simulink model "Correccion_Sist_Fisico"  (R2021a)
settings: Solver=VariableStepAuto  StartTime=0.0  StopTime=inf  RelTol=1e-3
values from neighbouring files (symbols this model uses):
  b_cx = 1*10^6    (= 1000000)    [parametros.m]
  b_cy = 1*10^7    (= 10000000)    [parametros.m]
  b_eq = (b_td+b_tm*(r_t^2))/r_td    (= 10803.6)    [parametros.m]
  b_eqh = 2*(b_hd+b_hm*(r_h^2))/r_hd    (= 23253.3333333)    [parametros.m]
  b_ha = b_eqh/r_h - n_h*w_posh*(J_eqh + 0.5*m_l_*r_hd)/r_h    [parametros.m]
  b_hb = 1*10^8    (= 100000000)    [parametros.m]
  b_hEb = 2.2*10^9    (= 2200000000)    [parametros.m]
  b_t = 90    [parametros.m]
  b_ta = n_t*w_post*(r_td*J_eqt/r_t) - r_td*b_eqt/r_t    [parametros.m]
  b_tb = 5*10^6    (= 5000000)    [parametros.m]
  b_tw = 3*10^3    (= 3000)    [parametros.m]
  b_wu = 150    [parametros.m]
  g = 9.80665    [parametros.m]
  H_c = 2.5    [parametros.m]
  J_eq = (J_td+J_tm_tb*(r_t^2))/r_td    (= 15000)    [parametros.m]
  J_eqh = 2*(J_hd_hEb+J_hm_hb*(r_h^2))/r_hd    (= 48853.3333333)    [parametros.m]
  K_cy = 1.8*10^9    (= 1800000000)    [parametros.m]
  K_hsa = -n_h*(w_posh^2)*(J_eqh + 0.5*m_l_*r_hd)/r_t    [parametros.m]
  K_hsia = -(w_posh^3)*(J_eqh + 0.5*m_l_*r_hd)/r_t    [parametros.m]
  K_tsa = n_t*(w_post^2)*J_eqt*r_td/r_t    [parametros.m]
  K_tsia = (w_post^3)*J_eqt*r_td/r_t    [parametros.m]
  K_tw = 4.8*10^5    (= 480000)    [parametros.m]
  k_wu = 2.36*10^8    (= 236000000)    [parametros.m]
  lh_inicial = 45-yl_inicial    (= 40)    [parametros.m]
  M_c_MAX = 50000 + M_s    (= 65000)    [parametros.m]
  M_real = 10000    [parametros.m]
  M_s = 15000    [parametros.m]
  M_t = 30000    [parametros.m]
  r_h = 22    [parametros.m]
  r_hd = 0.75    [parametros.m]
  r_t = 30    [parametros.m]
  r_td = 0.5    [parametros.m]
  T_hb_MAX = 5*10^4    (= 50000)    [parametros.m]
  T_hEb_MAX = 1.1*10^6    (= 1100000)    [parametros.m]
  T_hm_MAX = 2*10^4    (= 20000)    [parametros.m]
  T_s2 = 5e-3    (= 0.005)    [parametros.m]
  T_tb_MAX = 5*10^3    (= 5000)    [parametros.m]
  T_tm_MAX = 3*10^3    (= 3000)    [parametros.m]
  tau_hm = 1.0e-2    (= 0.01)    [parametros.m]
  tau_tm = 1.0e-2    (= 0.01)    [parametros.m]
  TensionMinima = (M_s*g/2)*0.5    (= 36774.9375)    [parametros.m]
  v_h_MAX_c = +1.5    (= 1.5)    [parametros.m]
  v_t_MAX = +4    (= 4)    [parametros.m]
  v_t_MIN = -4    [parametros.m]
  w_hm_min = pi/4    (= 0.785398163397)    [parametros.m]
  w_tm_min = pi/4    (= 0.785398163397)    [parametros.m]
  xt_inicial = -10    [parametros.m]
  Y_t0 = 45    [parametros.m]
  yl_inicial = 5    [parametros.m]
undefined symbols (not defined in the file or in its folder): DiscIntNeverNeededParam
libraries: simulink x10, dspstat3 x1, vrlib x1
(part 3 of 3)

== stateflow chart Correccion_Sist_Fisico/Chart ==
  note: ---> FINES DE CARRERA:
      |
      | 1. FIN DE CARRERA CARRO:
  state Nivel_1_Apagado
  note: ---> Si el Nivel 1 se encuentra apagodo deberia actuar el Nivel 0
  note: ---> Activado = Freno Energizado = Freno ABIERTO
  note: ---> Desactivado = Freno NO Energizado = Freno CERRADO
  state Nivel_1_Encendido
    state Sobrevelocidad [parallel]
      settings: executionOrder=12
      state CARRO [parallel]
        settings: executionOrder=2
        state Actualizacion_Vel_CARRO
          during:
          dx_t_SobreV = dx_t_ref_man;
        state Analisis_Sobrevelocidad
          entry:
          if (dx_t_ref_man>0)
          dx_t_SobreV = v_t_MAX;
          else
          dx_t_SobreV = v_t_MIN;
          end
        (default) -> Actualizacion_Vel_CARRO
        Actualizacion_Vel_CARRO -> Analisis_Sobrevelocidad : [abs(dx_t_ref_man) > v_t_MAX]
        Analisis_Sobrevelocidad -> Actualizacion_Vel_CARRO : [abs(dx_t_ref_man) <= v_t_MAX]
      state IZAJE [parallel]
        settings: executionOrder=1
        state Actualizacion_Vel_IZAJE
          during:
          dl_h_SobreV = dl_h_ref_man;
        state Analisis_Sobrevelocidad_Pos
          entry:
          dl_h_SobreV = v_h_MAXMIN;
        state Analisis_Sobrevelocidad_Neg
          entry:
          dl_h_SobreV = -v_h_MAXMIN;
        state BAJAR
          entry:
          dl_h_SobreV = v_h_MAX_c*0.1;
        (default) -> Actualizacion_Vel_IZAJE
        Actualizacion_Vel_IZAJE -> Analisis_Sobrevelocidad_Pos [order 1] : [(dl_h_ref_man > v_h_MAXMIN)  && ~sobrecarga ]
        Analisis_Sobrevelocidad_Pos -> Actualizacion_Vel_IZAJE : [(dl_h_ref_man <= v_h_MAXMIN) || sobrecarga ]
        Actualizacion_Vel_IZAJE -> Analisis_Sobrevelocidad_Neg [order 3] : [(dl_h_ref_man < -v_h_MAXMIN)   && ~sobrecarga ]
        Analisis_Sobrevelocidad_Neg -> Actualizacion_Vel_IZAJE : [(dl_h_ref_man >= -v_h_MAXMIN)  || sobrecarga ]
        Actualizacion_Vel_IZAJE -> BAJAR [order 2] : [sobrecarga]
        BAJAR -> Actualizacion_Vel_IZAJE : [~sobrecarga]
    state Fines_de_Carrera [parallel]
      settings: executionOrder=2
      state FIN_DE_CARRERA_CARRO [parallel]
        settings: executionOrder=1
        state Frenar
          entry:
          Detener_CarroFDC = 1;
        state MOVER_CARRO
          during:
          Detener_CarroFDC = 0;
        state No_Frenar
          entry:
          Detener_CarroFDC = 0;
        (default) -> Nivel_1_Encendido.Fines_de_Carrera.FIN_DE_CARRERA_CARRO.No_Frenar
        Nivel_1_Encendido.Fines_de_Carrera.FIN_DE_CARRERA_CARRO.Frenar -> Nivel_1_Encendido.Fines_de_Carrera.FIN_DE_CARRERA_CARRO.MOVER_CARRO [order 2] : [((dx_t_ref_man < 0 && Fin_Der_n) || (dx_t_ref_man > 0 && Fin_Izq_n))]
        Nivel_1_Encendido.Fines_de_Carrera.FIN_DE_CARRERA_CARRO.No_Frenar -> Nivel_1_Encendido.Fines_de_Carrera.FIN_DE_CARRERA_CARRO.Frenar : [Fin_Der_n || Fin_Izq_n]
        Nivel_1_Encendido.Fines_de_Carrera.FIN_DE_CARRERA_CARRO.MOVER_CARRO -> Nivel_1_Encendido.Fines_de_Carrera.FIN_DE_CARRERA_CARRO.Frenar : [(dx_t_ref_man >= 0 && Fin_Der_n) || (dx_t_ref_man <= 0 && Fin_Izq_n) || (~Fin_Der_n && ~Fin_Izq_n) ]
        Nivel_1_Encendido.Fines_de_Carrera.FIN_DE_CARRERA_CARRO.Frenar -> Nivel_1_Encendido.Fines_de_Carrera.FIN_DE_CARRERA_CARRO.No_Frenar [order 1] : [~Fin_Der_n && ~Fin_Izq_n]
      state FIN_DE_CARRERA_IZAJE [parallel]
        settings: executionOrder=2
        state Frenar
          entry:
          Detener_IzajeFDC = 1;
        state MOVER_IZAJE
          during:
          Detener_IzajeFDC = 0;
        state No_Frenar
          entry:
          Detener_IzajeFDC = 0;
        (default) -> Nivel_1_Encendido.Fines_de_Carrera.FIN_DE_CARRERA_IZAJE.No_Frenar
        Nivel_1_Encendido.Fines_de_Carrera.FIN_DE_CARRERA_IZAJE.Frenar -> Nivel_1_Encendido.Fines_de_Carrera.FIN_DE_CARRERA_IZAJE.MOVER_IZAJE [order 2] : [((dl_h_ref_man > 0 && Fin_Sup_n) || (dl_h_ref_man < 0 && Fin_Inf_n))]
        Nivel_1_Encendido.Fines_de_Carrera.FIN_DE_CARRERA_IZAJE.No_Frenar -> Nivel_1_Encendido.Fines_de_Carrera.FIN_DE_CARRERA_IZAJE.Frenar : [Fin_Sup_n || Fin_Inf_n]
        Nivel_1_Encendido.Fines_de_Carrera.FIN_DE_CARRERA_IZAJE.MOVER_IZAJE -> Nivel_1_Encendido.Fines_de_Carrera.FIN_DE_CARRERA_IZAJE.Frenar : [(dl_h_ref_man <= 0 && Fin_Sup_n) || (dl_h_ref_man >= 0 && Fin_Inf_n) || (~Fin_Sup_n && ~Fin_Inf_n) ]
        Nivel_1_Encendido.Fines_de_Carrera.FIN_DE_CARRERA_IZAJE.Frenar -> Nivel_1_Encendido.Fines_de_Carrera.FIN_DE_CARRERA_IZAJE.No_Frenar [order 1] : [~Fin_Sup_n && ~Fin_Inf_n]
    state Frenos [parallel]
      settings: executionOrder=4
      note: % Freno desactivado = Frenando
      state FRENO_CARRO [parallel]
        settings: executionOrder=1
        state No_Frenando
          entry:
          BRK_t = 1;
          Detener_CarroFR = 0;
        state Frenando
          entry:
          BRK_t = 0;
          Detener_CarroFR = 1;
        (default) -> Nivel_1_Encendido.Frenos.FRENO_CARRO.Frenando
        Nivel_1_Encendido.Frenos.FRENO_CARRO.No_Frenando -> Nivel_1_Encendido.Frenos.FRENO_CARRO.Frenando : [(abs(w_tm) < w_tm_min && Freno_Carro_Man) || (Emergencia == 2 && ~Salida_E_C) || sobrecarga || ( dx_t_ref == 0 && dx_t_SobreV == 0) ||  Detener_CarroFDC || (dx_t_ref * dx_t_ref_man < 0) ]
        Nivel_1_Encendido.Frenos.FRENO_CARRO.Frenando -> Nivel_1_Encendido.Frenos.FRENO_CARRO.No_Frenando : [Tmt_disp && ~Freno_Carro_Man && (Emergencia == 0 || Salida_E_C) && ~sobrecarga && ( dx_t_ref ~= 0 || dx_t_SobreV ~= 0) && ~Detener_CarroFDC && (dx_t_ref * dx_t_ref_man >= 0)]
      state FRENO_IZAJE [parallel]
        settings: executionOrder=2
        state No_Frenando
          entry:
          BRK_h = 1;
          Detener_IzajeFR = 0;
        state Frenando
          entry:
          BRK_h = 0;
          Detener_IzajeFR = 1;
        (default) -> Nivel_1_Encendido.Frenos.FRENO_IZAJE.Frenando
        Nivel_1_Encendido.Frenos.FRENO_IZAJE.No_Frenando -> Nivel_1_Encendido.Frenos.FRENO_IZAJE.Frenando : [(abs(w_hm) < w_hm_min && Freno_Izaje_Man) || (Emergencia == 3 && ~Salida_E_I)  || (sobrecarga && dl_h_ref <= 0) || ( dl_h_ref == 0 && dl_h_SobreV == 0) || Detener_IzajeFDC || ~Cable_Tenso || (45-l_h < y_obstaculo-0.15 && dl_h_ref_man >= 0) || (dl_h_ref * dl_h_ref_man < 0)]
        Nivel_1_Encendido.Frenos.FRENO_IZAJE.Frenando -> Nivel_1_Encendido.Frenos.FRENO_IZAJE.No_Frenando : [Tmh_disp && ~Freno_Izaje_Man && (Emergencia == 0 || Salida_E_I) && (~sobrecarga || sobrecarga && dl_h_ref > 0) && ( dl_h_ref ~= 0 || dl_h_SobreV ~= 0) && ~Detener_IzajeFDC && Cable_Tenso && (45-l_h >= y_obstaculo-0.15 || dl_h_ref_man < 0) && (dl_h_ref * dl_h_ref_man >= 0)]
      state FRENO_EMERGENCIA [parallel]
        settings: executionOrder=3
        state No_Frenando
          entry:
          BRK_hE = 1;
        state Frenando
          entry:
          BRK_hE = 0;
        (default) -> Nivel_1_Encendido.Frenos.FRENO_EMERGENCIA.Frenando
        Nivel_1_Encendido.Frenos.FRENO_EMERGENCIA.No_Frenando -> Nivel_1_Encendido.Frenos.FRENO_EMERGENCIA.Frenando : [~Grua_Encendida || (45-l_h < y_obstaculo-0.2 && dl_h_ref_man >= 0)]
        Nivel_1_Encendido.Frenos.FRENO_EMERGENCIA.Frenando -> Nivel_1_Encendido.Frenos.FRENO_EMERGENCIA.No_Frenando : [Grua_Encendida && (45-l_h > y_obstaculo-0.2 || dl_h_ref_man < 0)]
    state Sobrecarga [parallel]
      settings: executionOrder=7
      note: SI HAY SOBRECARGA SOLO SE PUEDE BAJAR MANUALMENTE
      state CON_SOBRECARGA
        entry:
        sobrecarga = 1;
      state SIN_SOBRECARGA
        entry:
        sobrecarga = 0;
      (default) -> SIN_SOBRECARGA
      SIN_SOBRECARGA -> CON_SOBRECARGA : [M_cX > M_c_MAX && MasaFija && TLK]
      CON_SOBRECARGA -> SIN_SOBRECARGA : [M_cX < M_c_MAX && MasaFija && ~TLK]
    state Twistlocks [parallel]
      settings: executionOrder=3
      note: SE ACTIVA EL TLK SI EL OPERARIO LO DESEA Y
          | ADEMAS LA TENSION EN EL CABLE ES 0 (spreader apoyado)
      state TLK_ABIERTO
        entry:
        TLK = 0;
        y_obstaculo = 0;
        during:
        y_obstaculo = Y_co;
      state TLK_CERRADO
        entry:
        TLK = 1;
        during:
        y_obstaculo = Y_co + 2.5;
      (default) -> TLK_ABIERTO
      TLK_CERRADO -> TLK_ABIERTO : [~Activar_TLK && ~Cable_Tenso && TLK]
      TLK_ABIERTO -> TLK_CERRADO : [Activar_TLK && ~Cable_Tenso && ~TLK]
    state Senal_Vida [parallel]
      settings: executionOrder=9
      state Pulso_alto
        entry:
        Vida=1;
      state Pulso_bajo
        entry:
        Vida=0;
      (default) -> Pulso_bajo
      Pulso_bajo -> Pulso_alto : after(500,msec)
      Pulso_alto -> Pulso_bajo : after(10,msec)
    state Deteccion_Cable_Flojo [parallel]
      settings: executionOrder=5
      state CABLE_TENSO
        entry:
        Cable_Tenso = 1;
      state CABLE_FLOJO
        entry:
        Cable_Tenso = 0;
      (default) -> CABLE_TENSO
      CABLE_FLOJO -> CABLE_TENSO : [dl_h_ref_man < 0 || F_hw > TensionMinima ]
      CABLE_TENSO -> CABLE_FLOJO : [dl_h_ref_man >= 0 && F_hw <= TensionMinima]
    state Control_De_Balanceo [parallel]
      settings: executionOrder=6
      state ACTIVADO
        entry:
        BAC = 1;
      state DESACTIVADO
        entry:
        BAC = 0;
      (default) -> DESACTIVADO
      ACTIVADO -> DESACTIVADO : [~Balanceo || Emergencia ~=0]
      DESACTIVADO -> ACTIVADO : [Balanceo && Emergencia == 0]
    state MOVER_GRUA_ESTADO_EMERGENCIA_IZAJE [parallel]
      settings: executionOrder=10
      state MOVER_IZAJE
        entry:
        Salida_E_I = 1;
      state EMERGENCIA_IZAJE
        entry:
        Salida_E_I = 0;
      state NORMAL
        entry:
        Salida_E_I = 0;
      (default) -> NORMAL
      EMERGENCIA_IZAJE -> Nivel_1_Encendido.MOVER_GRUA_ESTADO_EMERGENCIA_IZAJE.MOVER_IZAJE [order 2] : [(dl_h_ref_man > 0 && Fin_Sup_u) || (dl_h_ref_man < 0 && Fin_Inf_u)]
      NORMAL -> EMERGENCIA_IZAJE : [Emergencia == 3]
      EMERGENCIA_IZAJE -> NORMAL [order 1] : [Emergencia == 0]
      Nivel_1_Encendido.MOVER_GRUA_ESTADO_EMERGENCIA_IZAJE.MOVER_IZAJE -> EMERGENCIA_IZAJE : [(dl_h_ref_man <= 0 && Fin_Sup_u) || (dl_h_ref_man >= 0 && Fin_Inf_u) || Emergencia == 0]
    state MOVER_GRUA_ESTADO_EMERGENCIA_CARRO [parallel]
      settings: executionOrder=11
      state MOVER_CARRO
        entry:
        Salida_E_C = 1;
      state INICIO
        entry:
        Salida_E_C = 0;
      state ESPERA
        Salida_E_C = 0;
      (default) -> INICIO
      ESPERA -> Nivel_1_Encendido.MOVER_GRUA_ESTADO_EMERGENCIA_CARRO.MOVER_CARRO [order 2] : [(dx_t_ref_man < 0 && Fin_Der_u) || (dx_t_ref_man > 0 && Fin_Izq_u)]
      INICIO -> ESPERA : [Emergencia == 2]
      Nivel_1_Encendido.MOVER_GRUA_ESTADO_EMERGENCIA_CARRO.MOVER_CARRO -> ESPERA : [(dx_t_ref_man >= 0 && Fin_Der_u) || (dx_t_ref_man <= 0 && Fin_Izq_u) || Emergencia == 0]
      ESPERA -> INICIO [order 1] : [Emergencia == 0]
    state Modo [parallel]
      settings: executionOrder=8
      state MANUAL
        entry:
        Modo_Manual = 1;
        IteracionTerminada = 0;
        state Carro [parallel]
          settings: executionOrder=1
          state Operacion_Normal
            during:
            dx_t_ref = calcular_velocidad_maximaC(dx_t_SobreV);
          state sobrecarga_Carro
            entry:
            dx_t_ref = 0;
            calcular_velocidad_maximaC(0);
          state Analisis_FDC_D
            during:
            dx_t_ref = calcular_velocidad_maximaC(dx_t_SobreV*(50-x_td)/10);
          state Analisis_FDC_I
            during:
            dx_t_ref = calcular_velocidad_maximaC(dx_t_SobreV*(30+x_td)/10);
          state detener_carro
            entry:
            dx_t_ref = 0;
            calcular_velocidad_maximaC(0);
          (default) -> Nivel_1_Encendido.Modo.MANUAL.Carro.Operacion_Normal
          Analisis_FDC_D -> Nivel_1_Encendido.Modo.MANUAL.Carro.Operacion_Normal : [Detener_CarroFR || Detener_CarroFDC || dx_t_ref_man < 0]
          Nivel_1_Encendido.Modo.MANUAL.Carro.Operacion_Normal -> sobrecarga_Carro [order 1] : [sobrecarga]
          sobrecarga_Carro -> Nivel_1_Encendido.Modo.MANUAL.Carro.Operacion_Normal : [~sobrecarga]
          Nivel_1_Encendido.Modo.MANUAL.Carro.Operacion_Normal -> Analisis_FDC_D [order 3] : [x_td >=40 && dx_t_ref_man > 0 && ~Detener_CarroFR && ~Detener_CarroFDC && ~Fin_Der_n && ~Fin_Izq_n]
          Analisis_FDC_I -> Nivel_1_Encendido.Modo.MANUAL.Carro.Operacion_Normal : [Detener_CarroFR || Detener_CarroFDC || dx_t_ref_man > 0]
          Nivel_1_Encendido.Modo.MANUAL.Carro.Operacion_Normal -> detener_carro [order 2] : [Detener_CarroFR || Detener_CarroFDC ]
          Nivel_1_Encendido.Modo.MANUAL.Carro.Operacion_Normal -> Analisis_FDC_I [order 4] : [x_td <=-20 && dx_t_ref_man < 0 && ~Detener_CarroFR && ~Detener_CarroFDC]
          detener_carro -> Nivel_1_Encendido.Modo.MANUAL.Carro.Operacion_Normal : [~Detener_CarroFR  && ~Detener_CarroFDC ]
        state Izaje [parallel]
          settings: executionOrder=2
          note: dl_h_ref_man se refiere a longitud del cable. Si es >0, se tiene mayor longitud de cable y la carga baja. Si es <0 la longitud disminuye y la carga baja. El 5 en FDC_ARRIBA es una medida de seguridad. En estimacion de masa se limita la velocidad al 10%.
          state Operacion_Normal
            during:
            dl_h_ref = calcular_velocidad_maxima_I(dl_h_SobreV, MasaFija);
          state sobrecarga_Izaje
            during:
            if (dl_h_ref_man>0)
            dl_h_ref = calcular_velocidad_maxima_I(dl_h_SobreV, MasaFija);
            else
            dl_h_ref = 0;
            calcular_velocidad_maxima_I(0, MasaFija);
            end
          state Analisis_FDC_ARRIBA
            during:
            dl_h_ref = calcular_velocidad_maxima_I(dl_h_SobreV*(l_h-5)/5, MasaFija);
          state Analisis_FDC_ABAJO
            during:
            dl_h_ref = calcular_velocidad_maxima_I(dl_h_SobreV*(65-l_h)/10, MasaFija);
          state detener_Izaje
            entry:
            dl_h_ref = 0;
            calcular_velocidad_maxima_I(0, MasaFija);
          state Analisis_ESTIMACION_MASA
            during:
            dl_h_ref = calcular_velocidad_maxima_I(dl_h_SobreV, MasaFija)*0.1;
          state Analisis_OBSTACULO
            during:
            dl_h_ref = calcular_velocidad_maxima_I(dl_h_SobreV*(45-y_obstaculo-l_h+0.2)/5, MasaFija);
          (default) -> Nivel_1_Encendido.Modo.MANUAL.Izaje.Operacion_Normal
          Analisis_FDC_ARRIBA -> Nivel_1_Encendido.Modo.MANUAL.Izaje.Operacion_Normal : [Detener_IzajeFR || Detener_IzajeFDC || dl_h_ref_man > 0]
          Nivel_1_Encendido.Modo.MANUAL.Izaje.Operacion_Normal -> sobrecarga_Izaje [order 1] : [sobrecarga]
          Nivel_1_Encendido.Modo.MANUAL.Izaje.Operacion_Normal -> Analisis_FDC_ARRIBA [order 4] : [l_h <=10 && dl_h_ref_man < 0 && ~Detener_IzajeFR && ~Detener_IzajeFDC]
          sobrecarga_Izaje -> Nivel_1_Encendido.Modo.MANUAL.Izaje.Operacion_Normal : [~sobrecarga]
          Analisis_FDC_ABAJO -> Nivel_1_Encendido.Modo.MANUAL.Izaje.Operacion_Normal : [Detener_IzajeFR || Detener_IzajeFDC  || dl_h_ref_man < 0]
          Nivel_1_Encendido.Modo.MANUAL.Izaje.Operacion_Normal -> Analisis_FDC_ABAJO [order 5] : [l_h >=55 && dl_h_ref_man > 0 && ~Detener_IzajeFR && ~Detener_IzajeFDC]
          Analisis_ESTIMACION_MASA -> Nivel_1_Encendido.Modo.MANUAL.Izaje.Operacion_Normal : [MasaFija || sobrecarga || Detener_IzajeFR || Detener_IzajeFDC]
          Nivel_1_Encendido.Modo.MANUAL.Izaje.Operacion_Normal -> detener_Izaje [order 2] : [(Detener_IzajeFR || Detener_IzajeFDC) && ~sobrecarga]
          detener_Izaje -> Nivel_1_Encendido.Modo.MANUAL.Izaje.Operacion_Normal : [(~Detener_IzajeFR && ~Detener_IzajeFDC) || sobrecarga]
          Nivel_1_Encendido.Modo.MANUAL.Izaje.Operacion_Normal -> Analisis_ESTIMACION_MASA [order 6] : [~MasaFija && TLK && ~Detener_IzajeFR && ~Detener_IzajeFDC && Cable_Tenso]
          Analisis_OBSTACULO -> Nivel_1_Encendido.Modo.MANUAL.Izaje.Operacion_Normal : [Detener_IzajeFR || Detener_IzajeFDC  || dl_h_ref_man < 0]
          Nivel_1_Encendido.Modo.MANUAL.Izaje.Operacion_Normal -> Analisis_OBSTACULO [order 3] : [(y_obstaculo+5) >= (45-l_h) && dl_h_ref_man > 0 && ~Detener_IzajeFR && ~Detener_IzajeFDC]
      state AUTOMATICO
        entry:
        Modo_Manual = 0;
        esperando_estabilizacion=true;
        punto_muelle = [-20, 0];
        trayectoria = 0;
        punto_carga = [-10, 5];
        punto_descarga = [-15, 5];
        [contenedor_posiciones, y_max] = actualizar_contenedores(contenedor_pos_iniciales, -10, 10);
      (default) -> MANUAL
      MANUAL -> AUTOMATICO : [Cambiar_Modo && ~IteracionTerminada]
      AUTOMATICO -> MANUAL : [~Cambiar_Modo && IteracionTerminada || Emergencia || dx_t_ref_man ~= 0 || dl_h_ref_man ~= 0]
    state OBSTACULOS [parallel]
      entry:
      [contenedor_posiciones, y_max] = actualizar_contenedores(contenedor_pos_iniciales, -10, 10); % Pongo valor random para q me devuelva
      matriz_Y_co = calculo_matriz_yc0(contenedor_posiciones)                                                        % el y_max y no hacer otra funcion
      settings: executionOrder=1
      state ACTUALIZACION_CONTENEDORES [parallel]
        settings: executionOrder=1
        state Verificar
        state Carga
          entry:
          y_actual = pos_y_actual(l_h, TLK);
          [contenedor_posiciones, y_max] = actualizar_contenedores(contenedor_posiciones, x_td, y_actual);
          matriz_Y_co = calculo_matriz_yc0(contenedor_posiciones);
        state Descarga
          entry:
          % Por ahora no hace nada, va a servir para los otros modos
        (default) -> Verificar
        Verificar -> Carga [order 1] : [~Cable_Tenso &&  Activar_TLK && ~TLK ]
        Carga -> Verificar : [Cable_Tenso && MasaFija]
        Verificar -> Descarga [order 2] : [Cable_Tenso &&  ~Activar_TLK && TLK ]
        Descarga -> Verificar : [~Cable_Tenso]
      state CALCULAR_YCO [parallel]
        settings: executionOrder=2
        state Calculo_YC0
          during:
          Y_co = obtener_Y_c0(matriz_Y_co, x_td);
        (default) -> Calculo_YC0
  (default) -> Nivel_1_Apagado
  Nivel_1_Apagado -> Nivel_1_Encendido : [Alimentacion]
  Nivel_1_Encendido -> Nivel_1_Apagado : [~Alimentacion]
  data: dx_manual function_input; v_max_carro function_output; dh_manual function_input; v_max_izaje function_output; Enclave function_input; contenedor_pos function_output; contenedor_pos function_input; pos_x function_input; pos_y function_input; y_superior function_output; obstaculos function_input; punto_inicial function_input; punto_final function_input; Carga_Descarga_ function_input; perfil_trayectoria function_output; sx function_output; sy function_output; contenedor_pos function_output; contenedor_pos function_input; pos_x function_input; pos_y function_input; y_superior function_output; matriz_yc0 function_output; contenedor_pos function_input; matriz_yc0 function_input; yc0 function_output; xtd function_input; l function_input; tlk function_input; pos_y function_output; Alimentacion input; Fin_Der_n input; Fin_Izq_n input; Fin_Sup_n input; Fin_Inf_n input; BRK_t output; BRK_h output; BRK_hE output; Vida output size=1; Emergencia input; Grua_Encendida input; dx_t_ref_man input; dl_h_ref_man input; w_tm input; w_hm input; Freno_Carro_Man input; Freno_Izaje_Man input; Balanceo input; x_td input; l_h input; MasaFija input; Activar_TLK input; M_cX input; dx_t_ref output =0; dl_h_ref output =0; BAC output; TLK output size=1; v_t_MAX parameter; v_t_MIN parameter; Tmt_disp input; w_tm_min parameter; w_hm_min parameter; Tmh_disp input; F_hw input; v_h_MAX_c parameter; Modo_Manual output size=1; Detener_Carro local; Detener_Izaje local; Cable_Tenso local; dx_t_SobreV local =0; dl_h_SobreV local =0; sobrecarga local; M_c_MAX parameter; TensionMinima parameter; v_h_MAXMIN input; Detener_IzajeFDC local; Detener_CarroFDC local; Detener_CarroFR local; Detener_IzajeFR local; Fin_Sup_u input; Fin_Inf_u input; Cambio_Modo input; Fin_Izq_u input; Fin_Der_u input; Salida_E_C local; Salida_E_I local; bajar_sobrecarga local; y_obstaculo local; esperando_estabilizacion local; punto_limite local; punto_muelle local; trayectoria_y local; perfil_vel_x local; punto_inicial local; posicion_final local; perfil_vel_y local; Cambiar_Modo local; cant_puntos_discretizacion local; y_l local; y_sup local; it local; posicion_y_actual local size=1 =yl_inicial; y_max local; y_actual local; matriz_Y_co local size=1,16; contenedor_posiciones local size=18,16; contenedor_pos_iniciales input; Y_co output size=1
  function v_max_carro = calcular_velocidad_maximaC(dx_manual):
    | function v_max_carro = calcular_velocidad_maximaC(dx_manual)
    | 
    | %--------------------------------------------------------------------------%
    | %---------------------Declaracion variables PERSISTENT---------------------% 
    | %--------------------------------------------------------------------------%
    |             % --> Persistent: local variable in a function that retains its 
    |                             % value in memory between calls to the function
    |     persistent dx_t_ref_manual_anterior;
    |     a_max_carro = 1;     % m/s^2 (aceleracion max para el subsistema carro)
    |     dt = 0.02;           % 20 ms (tiempo de muestreo del statechart)
    |     
    | %--------------------------------------------------------------------------%
    | %------------------Inicialización de variables PERSISTENT------------------% 
    | %--------------------------------------------------------------------------%
    | 
    |     if isempty(dx_t_ref_manual_anterior)
    |         dx_t_ref_manual_anterior = 0;
    |     end
    |     
    | %--------------------------------------------------------------------------%
    | %-----------------------------Lógica principal-----------------------------%
    | %--------------------------------------------------------------------------%
    | % La idea es que el sistema siempre vaya a la maxima velocidad que pueda.
    | % Para eso se utiliza la aceleracion maxima para el subsistema carro en
    | % caso de que la velocidad de referencia no sea lo suficientemente grande.
    | % Si la velocidad supera la velocidad maxima, esta se limita al maximo
    | % permitido.
    |     if (dx_manual == 0)
    |         v_max_carro_aux = 0;
    |     else
    |         if abs(dx_manual) >= abs(dx_t_ref_manual_anterior)
    |             if dx_manual > 0                                                    % Aceleracion +
    |                 v_max = a_max_carro * dt + dx_t_ref_manual_anterior;
    |                 v_max_carro_aux = max(v_max, dx_manual);
    |             else                                                                % Aceleracion -
    |                 v_max = -a_max_carro * dt + dx_t_ref_manual_anterior;
    |                 v_max_carro_aux = min(v_max, dx_manual);
    |             end
    |         elseif dx_manual < dx_t_ref_manual_anterior                             % Desaceleracion -
    |             v_max = -a_max_carro * dt + dx_t_ref_manual_anterior;
    |             v_max_carro_aux = min(v_max, dx_manual);
    |         else                                                                    % Desaceleracion +
    |             v_max = a_max_carro * dt + dx_t_ref_manual_anterior;
    |             v_max_carro_aux = max(v_max, dx_manual);
    |         end
    | 
    |         if abs(v_max_carro_aux) > 4
    |             if v_max_carro_aux > 0
    |                 v_max_carro_aux = 4;
    |             else
    |                 v_max_carro_aux = -4;
    |             end
    |         end
    |     end
    |     v_max_carro = v_max_carro_aux;
    | 
    |     dx_t_ref_manual_anterior = v_max_carro;
    | end
  function v_max_izaje =   calcular_velocidad_maxima_I(dh_manual, Enclave):
    | function v_max_izaje =   calcular_velocidad_maxima_I(dh_manual, Enclave) % CT es Cable Tenso
    | 
    | %--------------------------------------------------------------------------%
    | %---------------------Declaracion variables PERSISTENT---------------------% 
    | %--------------------------------------------------------------------------%
    |             % --> Persistent: local variable in a function that retains its 
    |                             % value in memory between calls to the function
    |     persistent dy_href_manual_ant;
    |     persistent a_max_y;  % m/s^2
    |     persistent dt;       % 20 ms (tiempo de muestreo del statechart)
    |     
    | %--------------------------------------------------------------------------%
    | %------------------Inicialización de variables PERSISTENT------------------% 
    | %--------------------------------------------------------------------------%
    | 
    |     if isempty(dy_href_manual_ant)
    |         dy_href_manual_ant = 0;
    |     end
    |     if isempty(a_max_y)
    |         a_max_y = 0.75;  % m/s^2
    |     end
    |     if isempty(dt)
    |         dt = 0.02;       % 20 ms (tiempo de muestreo del statechart)
    |     end
    |     
    | %--------------------------------------------------------------------------%
    | %-----------------------------Lógica principal-----------------------------%
    | %--------------------------------------------------------------------------%
    | % La idea es que el sistema siempre vaya a la maxima velocidad que pueda.
    | % Para eso se utiliza la aceleracion maxima para el subsistema carro en
    | % caso de que la velocidad de referencia no sea lo suficientemente grande.
    | % Si la velocidad supera la velocidad maxima, esta se limita al maximo
    | % permitido.
    |     if (dh_manual ==0)
    |         v_max_izaje_aux = 0;
    |     else
    |         if abs(dh_manual) >= abs(dy_href_manual_ant)
    |             if dh_manual > 0
    |                 v_max = a_max_y * dt + dy_href_manual_ant;
    |                 v_max_izaje_aux = max(v_max, dh_manual);
    |             else
    |                 v_max = -a_max_y * dt + dy_href_manual_ant;
    |                 v_max_izaje_aux = min(v_max, dh_manual);
    |             end
    |         else
    |             if dh_manual < dy_href_manual_ant
    |                 v_max = -a_max_y * dt + dy_href_manual_ant;
    |                 v_max_izaje_aux = min(v_max, dh_manual);
    |             else
    |                 v_max = a_max_y * dt + dy_href_manual_ant;
    |                 v_max_izaje_aux = max(v_max, dh_manual);
    |             end
    |         end
    | 
    |         if Enclave == 1      % Hay carga, velocidad maxima 1.5 m/s
    |             if abs(v_max_izaje_aux) > 1.5
    |                 if v_max_izaje_aux > 0
    |                     v_max_izaje_aux = 1.5;
    |                 else
    |                     v_max_izaje_aux = -1.5;
    |                 end
    |             end
    |         else                % No hay carga, velocidad maxima 3 m/s
    |             if abs(v_max_izaje_aux) > 3
    |                 if v_max_izaje_aux > 0
    |                     v_max_izaje_aux = 3;
    |                 else
    |                     v_max_izaje_aux = -3;
    |                 end
    |             end
    |         end
    |     end
    |     v_max_izaje = v_max_izaje_aux;
    |     dy_href_manual_ant = v_max_izaje;
    | 
    | end
  function [contenedor_pos, y_superior] = actualizar_contenedores(contenedor_pos, pos_x, pos_y):
    | function [contenedor_pos, y_superior] = actualizar_contenedores(contenedor_pos, pos_x, pos_y)
    |     for columna = 1:size(contenedor_pos, 2)
    |         cantidad_contenedores_columna = sum(contenedor_pos(:,columna));
    |         if cantidad_contenedores_columna ~= 0 % Es decir si quedan contenedores en esa columna
    |             pos_x_izq_contenedor = 2.5 + (columna - 1) * 3;
    |             pos_x_der_contenedor = pos_x_izq_contenedor + 2.5;
    |             tolerancia = 0.2;
    |             pos_y_superior_contenedor = cantidad_contenedores_columna * 2.5 + tolerancia;
    |             if pos_x > pos_x_izq_contenedor && pos_x < pos_x_der_contenedor && pos_y < pos_y_superior_contenedor 
    |                 contenedor_pos(cantidad_contenedores_columna, columna) = 0;
    |                 break;
    |             end
    |         end
    |     end
    |     unos_por_columna = sum(contenedor_pos); % Me da la suma de cada columna
    |     max_contenedores = max(unos_por_columna); % Busco el máximo de la suma de cada columna
    |     
    |     coef_seguridad = 5;
    |     y_superior = max_contenedores*2.5 + coef_seguridad;
    | end
  function [perfil_trayectoria, sx, sy]  = generar_Trayectoria2(obstaculos, punto_inicial, punto_final, Carga_Descarga_):
    | function [perfil_trayectoria, sx, sy]  = generar_Trayectoria2(obstaculos, punto_inicial, punto_final, Carga_Descarga_) 
    | 
    | %===================================================PERFIL DE VELOCIDAD
    |     %________________Aceleraciones y velocidades
    |     
    | 
    |     perfil_vel_x = [0];
    |     perfil_vel_y = [];
    |     
    |     amax_Y = 0.75;
    |     vmax_Y = 3;
    |     vmax_X = 4;
    |     amax_X = 1;
    |     
    |     
    | %===================================================PERFIL DE TRAYECTORIA
    |     %________________Definir inicio contenedores y el factor de seguridad
    |     factor_seguridad = 3;
    |     inicio_contenedores = [2.5, -20];
    |     contador = 0;
    |     
    |     separacion_contenedores = 0.5;
    |     pared_barco = zeros(length(obstaculos(:,1)),1);
    |     pared_barco(1:2, 1) = [1, 1];
    |     obstaculos = [pared_barco, obstaculos];
    |     
    |     %________________Definir las dimensiones de los contenedores y el incremento de altura y posición
    |     ancho_contenedor = 2.5;
    |     alto_contenedor = 2.5;
    |     incremento_altura = 2;
    |     incremento_posicion = 0.625;
    |     incremento_altura_vuelta = 1;
    |     incremento_altura_bajada = 3;
    |     punto_final_aux = 0;
    |     
    |     
    |     % Inicializar el perfil de trayectoria como un vector vacío
    |     perfil_trayectoria = [punto_inicial];
    | 
    |     % Verificar cual es el obstáculo más alto
    |     obstaculo_mas_alto = max(sum(obstaculos, 1));
    | 
    |     % Calcular la altura del obstáculo más alto en metros
    |     if Carga_Descarga_ == 0
    |         altura_obstaculo_mas_alto = obstaculo_mas_alto * alto_contenedor + factor_seguridad*2 + inicio_contenedores(1, 2);
    |     else
    |         posicion = encontrar_posicion(punto_inicial, obstaculos);
    |         if posicion > 1
    |             contenedores_por_fila = cant_contenedores(obstaculos(:,posicion-1));
    |             altura_obstaculo_mas_alto = contenedores_por_fila * alto_contenedor + factor_seguridad*2 + inicio_contenedores(1, 2);
    |         elseif posicion == 1
    |             contenedores_por_fila = cant_contenedores(obstaculos(:,posicion+1));
    |             altura_obstaculo_mas_alto = contenedores_por_fila * alto_contenedor + factor_seguridad*2 + inicio_contenedores(1, 2);
    |         else
    |             altura_obstaculo_mas_alto = 7;
    |         end
    |     end
    | 
    |     if (punto_inicial(1, 1) < punto_final(1,1))
    |         disp('hola')
    |         punto_final = modificacion_punto_final(obstaculos,punto_final,  ancho_contenedor,alto_contenedor, factor_seguridad, separacion_contenedores);
    |     
    |         % Buscar una línea que una el punto inicial con un punto P2 ubicado en x en la pared del barco y con una altura igual a la del obstáculo más alto
    |         P2 = [0 + ancho_contenedor/2, altura_obstaculo_mas_alto]
    | 
    |         % Verificar si la línea colisiona con el perfil de obstáculos
    |         
    |         
    |         dy = P2(1,2) - punto_inicial(1,2);
    |         dx = P2(1,1) - punto_inicial(1,1);
    |         Tx1 = vmax_X/amax_X                                                 % TIEMPO HASTA VELOCIDAD MAX
    |         Tx3 = (abs(dx) - 0.5*(Tx1^2)*amax_X)/vmax_X
    |         if (Tx3>0)
    |             Tx = Tx1 + Tx3;
    |         else
    |             Tx = Tx1;
    |         end
    |         Ty1 = vmax_Y/amax_Y;
    |         Ty3 = (abs(dy) - 2*0.5*(Ty1^2)*amax_Y)/vmax_Y;
    |         Ty = 2*Ty1 + Ty3  % TIEMPO PERFIL TRAPEZOIDAL
    |         Tx
    |         if(Tx == Ty)
    |             disp('');
    |             colision = verificar_colision_SUBIDA_IDA(obstaculos, punto_inicial, P2, ancho_contenedor, alto_contenedor, factor_seguridad);
    |         else                                                                % SIEMPRE TY VA A SER MAS GRANDE
    |             T = Ty - Tx
    |             
    |             if T <= Ty1
    |                 dy_aux  = 0.5*amax_Y*(T^2);
    |             elseif T > Ty1 && T<= Ty1 + Ty3
    |                 dy_aux = 0.5*amax_Y*(Ty1^2) + vmax_Y*(T-Ty1);
    |             else 
    |                 dy_aux = 0.5*amax_Y*(Ty1^2) + vmax_Y*(Ty3) + vmax_Y*(T - Ty1 - Ty3) - 0.5*amax_Y*((T - Ty1 - Ty3)^2);
    |             end
    |             colision = verificar_colision_SUBIDA_IDA(obstaculos, punto_inicial, P2, ancho_contenedor, alto_contenedor, factor_seguridad);
    |             
    |             if true
    |                 perfil_vel_y = [perfil_vel_y, linspace(0, vmax_Y, Ty1/0.005), linspace(vmax_Y, vmax_Y, Ty3/0.005), linspace(vmax_Y, 0, Ty1/0.005)];
    |                 if (Tx3>=0)
    |                     disp('Hola')
    |                      perfil_vel_x = [perfil_vel_x, linspace(0, 0, T/0.005), linspace(0, vmax_X, (Tx1)/0.005), linspace(vmax_X, vmax_X, (Tx3)/0.005)];
    |                 else
    |                      perfil_vel_x = [perfil_vel_x, linspace(0, 0, T/0.005), linspace(0, vmax_X, (Tx)/0.005)];
    |                 end
    |                 
    |                 sx = punto_inicial(1,1);
    |                 sy = punto_inicial(1,2);
    |                 for ii = 2: length(perfil_vel_y)
    |                     if 0.005*ii <= (Ty1)
    |                         sy(ii) = sy(ii-1) + 0.5 * amax_Y * (0.005*ii - 0.005*(ii-1))^2 + perfil_vel_y(ii-1)*(0.005*ii-0.005*(ii-1));
    |                     elseif 0.005*ii > (Ty1) && 0.005*ii <= (Ty1 + Ty3)
    |                         sy(ii) = sy(ii-1) + vmax_Y*(0.005*ii-0.005*(ii-1));
    |                     else
    |                         sy(ii) = sy(ii-1) - 0.5 * amax_Y * (0.005*ii - 0.005*(ii-1))^2 + perfil_vel_y(ii-1)*(0.005*ii-0.005*(ii-1));
    |                     end
    |                     if 0.005*ii <= T
    |                         sx(ii) = sx(1);
    |                     else
    |                         sx(ii) = sx(ii-1) + 0.5 * amax_X * (0.005*ii - 0.005*(ii-1))^2 + perfil_vel_x(ii-1)*(0.005*ii-0.005*(ii-1)); 
    |                     end
    |                 end
    |             end
    |         end
    | 
    |         % Si hay colisión, elevar el punto inicial 2 metros y volver a buscar la línea
    |         while colision
    |             contador = 1;
    |             punto_inicial(2) = punto_inicial(2) + incremento_altura;
    |             colision = verificar_colision_SUBIDA_IDA(obstaculos, punto_inicial, P2, ancho_contenedor, alto_contenedor, factor_seguridad);
    |             
    |         end
    |         % Agregar el punto al perfil de trayectoria
    |         if (contador ~= 0)
    |             perfil_trayectoria = [perfil_trayectoria; punto_inicial; P2];
    |             contador = 0;
    |         else
    |             perfil_trayectoria = [perfil_trayectoria; P2];
    |         end
    |         % Buscar una línea que una el punto P2 con el punto final
    |         colision = verificar_colision_BAJADA_IDA(obstaculos, P2, punto_final, ancho_contenedor, alto_contenedor, factor_seguridad);
    | 
    |         % Si hay colisión, mover el punto P2 2 metros en el eje x y buscar una nueva línea
    |         punto_final_aux = punto_final + [0, 1.5];
    |         i_ = 1;
    |         
    |         while colision
    |             contador = 1;
    |             if (i_ == 4 || i_ == 7 || i_ ==10 || i_ ==13 || i_ ==16 || i_ ==19 || i_ ==21)
    |                 P2(1) = P2(1) + 0.5;
    |             else
    |                 P2(1) = P2(1) + incremento_posicion;
    |             end
    |             i_ = i_+1;
    |             punto_final_aux(2) = punto_final_aux(2) + 0.5;
    |             colision = verificar_colision_BAJADA_IDA(obstaculos, P2, punto_final_aux, ancho_contenedor, alto_contenedor, factor_seguridad);
    |         end
    | 
    |         % Agregar la línea al perfil de trayectoria
    |         if (contador ~= 0)
    |             perfil_trayectoria = [perfil_trayectoria; P2; punto_final_aux; punto_final];
    |             contador = 0;
    |         else
    |             perfil_trayectoria = [perfil_trayectoria;punto_final_aux; punto_final];
    |         end
    |         disp(punto_final)
    |         if(punto_final(1) == -10 && punto_final(2) == 10.5)
    |             disp('adentro x2')
    |             perfil_trayectoria = [punto_inicial;punto_inicial + [0, altura_obstaculo_mas_alto]; punto_final]
    |         end
    |         t = linspace(0, Ty, Ty/0.005);
    |         length(t)
    |         length(perfil_vel_x)
    |         figure(4)
    |         plot(t, perfil_vel_y)
    |         figure(5)
    |         plot(t, perfil_vel_x)
    |         
    |     else
    |         % Buscar una línea que una el punto inicial con un punto P2 ubicado en x en el primer contenedor y con una altura igual a la del obstáculo más alto
    |         P2 = [punto_inicial(1,1) - ancho_contenedor, altura_obstaculo_mas_alto];
    |         punto_inicial(1,1);
    | 
    |         % Verificar si la línea colisiona con el perfil de obstáculos
    |         colision = verificar_colision_SUBIDA_VUELTA(obstaculos, punto_inicial, P2, ancho_contenedor, alto_contenedor, factor_seguridad);
    | 
    |         % Si hay colisión, elevar el punto inicial 2 metros y volver a buscar la línea
    |         while colision
    |             
    |             contador = 1;
    |             punto_inicial(2) = punto_inicial(2) + incremento_altura_vuelta;
    |             colision = verificar_colision_SUBIDA_VUELTA(obstaculos, punto_inicial, P2, ancho_contenedor, alto_contenedor, factor_seguridad);
    |         end
    |         
    |         % Agregar el punto al perfil de trayectoria
    |         if (contador ~= 0)
    |             perfil_trayectoria = [perfil_trayectoria; punto_inicial; P2];
    |             contador = 0;
    |         else
    |             perfil_trayectoria = [perfil_trayectoria; P2];
    |         end
    |         % Buscar una línea que una el punto P2 con el punto final
    |         colision = verificar_colision_BAJADA_VUELTA(obstaculos, P2, punto_final, ancho_contenedor, alto_contenedor, factor_seguridad);
    | 
    |         % Si hay colisión, mover el punto P2 2 metros en el eje x y buscar una nueva línea
    |         punto_final_aux = punto_final;
    |         while colision
    |             contador = 1;
    |             P2(1) = P2(1) - incremento_posicion;
    |             punto_final_aux(2) = punto_final(2) + incremento_altura_bajada;
    |             colision = verificar_colision_BAJADA_VUELTA(obstaculos, P2, punto_final, ancho_contenedor, alto_contenedor, factor_seguridad);
    |             
    |         end
    | 
    |         % Agregar la línea al perfil de trayectoria
    |         if (contador ~= 0)
    |             perfil_trayectoria = [perfil_trayectoria; P2;punto_final_aux; punto_final];
    |             contador = 0;
    |         else
    |             perfil_trayectoria = [perfil_trayectoria; punto_final];
    |         end
    |     end
    |     %plot(perfil_trayectoria(:, 1),perfil_trayectoria(:, 2), 'b');
    |     %perfil_trayectoria = perfil_trayectoria';
    | %_____________________________________________________________________________________________________________________
    | %___________________________________________________FUNCIONES_________________________________________________________
    | %_____________________________________________________________________________________________________________________
    | 
    | %===================================================PERFIL DE TRAYECTORIA
    |     % Definir una función auxiliar para verificar la colisión entre una línea y el perfil de obstáculos
    |     function colision = verificar_colision_SUBIDA_IDA(obstaculos, punto_a, punto_b, ancho_contenedor, alto_contenedor, factor_seguridad)
    |         % Calcular la ecuación de la recta que pasa por los dos puntos
    |         m = (punto_b(2) - punto_a(2)) / (punto_b(1) - punto_a(1));      % Pendiente de la recta
    |         b = punto_a(2) - m * punto_a(1);
    | 
    |         % Inicializar la variable de colisión como falsa
    |         colision = false;
    | 
    |         % Recorrer las columnas de la matriz de obstáculos
    |         % Calcular la posición x del contenedor
    |         x = 0 - factor_seguridad;                                       % En realidad es inicio_contenedor pero tiene el mismo valor
    | 
    |         % Calcular la posición y de la recta en esa posición x
    |         y = m * x + b;
    | 
    |         % Recorrer las filas de la matriz de obstáculos
    |         y_contenedor = cant_contenedores(obstaculos(:,1)) * alto_contenedor + factor_seguridad - 20;
    |         if y <= y_contenedor
    |             % Si es así, hay colisión
    |             colision = true;
    |         end
    |     end
    |     
    |     function colision = verificar_colision_BAJADA_IDA(obstaculos, punto_a, punto_b, ancho_contenedor, alto_contenedor, factor_seguridad)
    |         % Calcular la ecuación de la recta que pasa por los dos puntos
    |         m = (punto_b(2) - punto_a(2)) / (punto_b(1) - punto_a(1));      % Pendiente de la recta
    |         b = punto_a(2) - m * punto_a(1);
    | 
    |         % Inicializar la variable de colisión como falsa
    |         colision = false;
    | 
    |         % Recorrer las columnas de la matriz de obstáculos
    |         for i = 1:size(obstaculos, 2)-1
    |             % Calcular la posición x del contenedor
    |             
    |             x = (ancho_contenedor)*(i+1) + factor_seguridad/2 + 0.5*(i-1);
    |             x_real = (ancho_contenedor)*(i+1) + 0.5*(i-1);
    |   
    |             % Calcular la posición y de la recta en esa posición x
    |             y = m * x + b;
    | 
    |             % Recorrer las filas de la matriz de obstáculos
    |             y_contenedor = cant_contenedores(obstaculos(:, i+1)) * alto_contenedor + factor_seguridad -20;
    | 
    | 
    |             if y <= y_contenedor && x <= (punto_b(1)+ 0)
    |                 % Si es así, hay colisión
    |                 disp('colision') 
    |                 colision = true;
    |                 % Salir del bucle
    |                 break;
    |             end
    |         end
    |     end
    | 
    | % Definir una función auxiliar para verificar la colisión entre una línea y el perfil de obstáculos
    |     function colision = verificar_colision_SUBIDA_VUELTA(obstaculos, punto_a, punto_b, ancho_contenedor, alto_contenedor, factor_seguridad)
    |         % Calcular la ecuación de la recta que pasa por los dos puntos
    |         m = (punto_b(2) - punto_a(2)) / (punto_b(1) - punto_a(1));      % Pendiente de la recta
    |         b = punto_a(2) - m * punto_a(1);
    | 
    |         % Inicializar la variable de colisión como falsa
    |         colision = false;
    | 
    |         for i = 1:size(obstaculos, 2)-1
    |             % Calcular la posición x del contenedor
    |             
    |             x = (ancho_contenedor)*(i+1) + 1 + 0.5*(i-1);
    |   
    |             % Calcular la posición y de la recta en esa posición x
    |             y = m * x + b;
    | 
    |             % Recorrer las filas de la matriz de obstáculos
    |             y_contenedor = cant_contenedores(obstaculos(:, i+1)) * alto_contenedor + factor_seguridad/2 -20;
    | 
    |             if y <= y_contenedor && x <= (punto_a(1)+ 0)
    |                 % Si es así, hay colisión
    |                 colision = true;
    |                 % Salir del bucle
    |                 break;
    |             end
    |         end
    |     end
    |     
    |     function colision = verificar_colision_BAJADA_VUELTA(obstaculos, punto_a, punto_b, ancho_contenedor, alto_contenedor, factor_seguridad)
    |         % Calcular la ecuación de la recta que pasa por los dos puntos
    |         m = (punto_b(2) - punto_a(2)) / (punto_b(1) - punto_a(1)) ;     % Pendiente de la recta
    |         b = punto_a(2) - m * punto_a(1);
    |         % Inicializar la variable de colisión como falsa
    |         colision = false;
    | 
    |         % Recorrer las columnas de la matriz de obstáculos
    |         for i = 1:size(obstaculos, 2)
    |             % Calcular la posición x del contenedor
    |             x = ancho_contenedor*i - factor_seguridad - ancho_contenedor;                                     
    | 
    |             % Calcular la posición y de la recta en esa posición x
    |             %disp('--')
    |             y = m * x + b;
    | 
    |             % Recorrer las filas de la matriz de obstáculos
    |             y_contenedor = cant_contenedores(obstaculos(:, i)) * alto_contenedor + factor_seguridad -20;
    |             
    |             if y <= y_contenedor
    |                 % Si es así, hay colisión
    |                 colision = true;
    |                 % Salir del bucle
    |                 break;
    |             end
    |             
    |         end
    |     end
    | 
    | 
    |     function contenedores_por_fila = cant_contenedores(fila)
    |         contenedores_por_fila = 0;
    |         for i = 1:length(fila)
    |             if fila(i) == 1
    |                 contenedores_por_fila = contenedores_por_fila + 1;
    |             end
    |         end
    |     end
    | 
    | 
    |     function punto_final_modificado = modificacion_punto_final(obstaculos,punto_final,  ancho_contenedor, alto_contenedor, factor_seguridad, separacion_contenedores)
    |         punto_final_modificado = [0, 0];
    |         obstaculos = obstaculos(:, 2:end);
    |         for i = 1: length(obstaculos(1,:))
    |             if(obstaculos(1,i) == 1)
    |                 if i ~= 1
    |                     x_izquierdo = ancho_contenedor*(i) + separacion_contenedores*(i-1);
    |                     x_derecho = ancho_contenedor*i + ancho_contenedor + separacion_contenedores*(i-1);
    |                 else
    |                     x_izquierdo = ancho_contenedor*i;
    |                     x_derecho = ancho_contenedor*i + ancho_contenedor;
    |                 end
    |                 if (punto_final(1) >= x_izquierdo && punto_final(1) <= x_derecho)
    |                     punto_final_modificado(1) = x_izquierdo + ancho_contenedor/2;
    | 
    |                     y_contenedor = cant_contenedores(obstaculos(:,i)) * alto_contenedor + factor_seguridad - 20;
    |                     if (punto_final(2) < y_contenedor)
    |                         punto_final_modificado(2) = y_contenedor;
    |                     else 
    |                         punto_final_modificado(2) = punto_final(2);
    |                     end
    |                     break;
    |                 else
    |                     punto_final_modificado(1) = punto_final(1);
    |                     y_contenedor = cant_contenedores(obstaculos(:,i)) * alto_contenedor + factor_seguridad - 20;
    |                     if (punto_final(2) < y_contenedor)
    |                         punto_final_modificado(2) = y_contenedor;
    |                     else 
    |                         punto_final_modificado(2) = punto_final(2);
    |                     end
    |                 end                                
    |             end
    |         end  
    |         
    |     end
    | 
    |     function posicion = encontrar_posicion(punto_inicial, obstaculos)
    |         posicion = 0;
    |         for j = 1:size(obstaculos, 2)-1
    |             % Calcular la posición x del contenedor
    |             ancho = 2.5;
    |             
    |             x_real_izq = (ancho)*(j) + 1 + 0.5*(j-1);
    |             x_real_der = (ancho)*(j+1) + 0.5*(j-1);
    |             
    |             if punto_inicial(1) > x_real_izq
    |                 posicion = posicion + 1;
    |                 if punto_inicial(1) < x_real_der
    |                     break;
    |                 end
    |             end
    |         end
    |     end
    | 
    | %===================================================PERFIL DE VELOCIDAD
    |     function perfil_vel = obtener_perfil_vel(puntos, puntos_aux, tipo, parametros)
    |         perfil_vel = [
    |             0; 
    |             0];
    |         t_ant = 0;
    |         for i = 1:numel(puntos)-1
    |             t1 = obtener_tiempo_espera(i, puntos, tipo, parametros);
    |             if tipo == 'x'
    |                 t2 = obtener_tiempo_espera(i, puntos_aux, 'y', parametros);
    |             else
    |                 t2 = obtener_tiempo_espera(i, puntos_aux, 'x', parametros);
    |             end
    | 
    |             if t1 >= t2
    |                 v_max = parametros.(tipo).v_max;
    |                 a_max = parametros.(tipo).a_max;
    |                 perfil_velocidad = obtener_perfil_vel_aux(i, puntos, puntos_aux, tipo, t_ant, v_max, a_max);
    |             else
    |                 v = 2 * abs(puntos(i+1) - puntos(i)) / t2;
    |                 a = v / (t2 / 2);
    |                 perfil_velocidad = obtener_perfil_vel_aux(i, puntos, puntos_aux, tipo, t_ant, v, a);
    |             end
    |             perfil_vel = [perfil_vel, perfil_velocidad];
    |             t_ant = perfil_vel(1, end); 
    |         end
    |     end
    | 
    | 
    | %_____________________________________________________________________________________________________________________
    | %__________________________________________________END FUNCIONES______________________________________________________
    | %_____________________________________________________________________________________________________________________
    | 
    | 
    | end
  function [contenedor_pos, y_superior] = actualizar_contenedores(contenedor_pos, pos_x, pos_y):
    | function [contenedor_pos, y_superior] = actualizar_contenedores(contenedor_pos, pos_x, pos_y)
    |     for columna = 1:size(contenedor_pos, 2)
    |         cantidad_contenedores_columna = sum(contenedor_pos(:,columna));
    |         if cantidad_contenedores_columna ~= 0 % Es decir si quedan contenedores en esa columna
    |             pos_x_izq_contenedor = 2.5 + (columna - 1) * 3;
    |             pos_x_der_contenedor = pos_x_izq_contenedor + 2.5;
    |             tolerancia = 0.2;
    |             pos_y_superior_contenedor = cantidad_contenedores_columna * 2.5 + tolerancia;
    |             if pos_x > pos_x_izq_contenedor && pos_x < pos_x_der_contenedor && pos_y < pos_y_superior_contenedor 
    |                 contenedor_pos(cantidad_contenedores_columna, columna) = 0;
    |                 break;
    |             end
    |         end
    |     end
    |     unos_por_columna = sum(contenedor_pos); % Me da la suma de cada columna
    |     max_contenedores = max(unos_por_columna); % Busco el máximo de la suma de cada columna
    |     
    |     coef_seguridad = 5;
    |     y_superior = max_contenedores*2.5 + coef_seguridad;
    | end
  function matriz_yc0 = calculo_matriz_yc0(contenedor_pos):
    | function matriz_yc0 = calculo_matriz_yc0(contenedor_pos)
    |     cant_columnas = size(contenedor_pos, 2);
    |     matriz_yc0 = zeros(1,cant_columnas);
    |     for columna = 1:cant_columnas
    |         cantidad_contenedores_columna = sum(contenedor_pos(:,columna));
    |         matriz_yc0(1,columna) = cantidad_contenedores_columna * 2.5 - 20; % -20 es la posición donde arrancan los contenedores a apoyarse
    |     end
    | end
  function yc0 = obtener_Y_c0(matriz_yc0, xtd):
    | function yc0 = obtener_Y_c0(matriz_yc0, xtd)
    |     yc0 = 0;
    |     if xtd >= 2.5 && xtd <= 48
    |         % 2.5 es donde empiezan los contenedores
    |         % 48 sería 3 (que es la distancia desde la parte izq del contenedor y la izq del siguiente)
    |         % por 16 columnas de contenedores
    |         coef_seguridad = 0.5;
    |         yc0 = matriz_yc0(1,ceil(xtd/3)) + coef_seguridad;
    |     end
    | end
  function pos_y = pos_y_actual(l, tlk):
    | function pos_y = pos_y_actual(l, tlk)
    |     if tlk
    |         pos_y=45-l-2.5;
    |     else
    |         pos_y=45-l;
    |     end
    | end
